simulink library "dsdc"  (Simulink 8.1)
settings: Solver=ode1  StartTime=0.0  StopTime=Inf  FixedStep=0.001  RelTol=1e-3
PostLoadFcn:
  | , if any(exist('dsrtsu_mdlpostloadfcn', 'file') == [2, 3, 6]), try dsrtsu_mdlpostloadfcn('Execute', bdroot); catch fprintf('Error in PostLoadFcn (dsrtsu_mdlpostloadfcn) for model "%s":\n %s\n', bdroot, lasterr); end, end,
undefined symbols (not defined in the file or in its folder): KJUD_EarlyTtcDelay_ms, KJUD_LateTtcDelay_ms, KJUD_NormalTtcDelay_ms
settings Model: DSRTSU_INTERNAL_RTI_VER=450  DSRTSU_INTERNAL_RTI_TYPE=rti1401  RTICANMMDATA=struct('GeneralSetupData',struct('modelroot','C:\Users\idiada\Desktop\HAITEC_Taiwan\trunk\AdasDragon\software\sw_development\arch\app\jud','generalsettings',struct('filesettings',struct('destfolder',struct('Name','RTICANMM_FILES','Check',1),'buildfolder',struct('Name','.','Check',1),'AbsDestfolder',struct('Name','C:\Users\idiada\Desktop\HAITEC_Taiwan\trunk\AdasDragon\software\sw_development\arch\app\jud\RTICANMM_FILES'),'AbsBuildfolder',struct('Name','C:\Users\idiada\Desktop\HAITEC_Taiwan\trunk\AdasDragon\software\sw_development\arch\app\jud'))),'options',struct('addpaths',1,'rmpaths',1,'addtrcexclusion',logical(1),'cannavigator',struct('checkmonitoring',0),'show_usrtrc',0,'use_usrtrc',0),'advanced',struct('options',[1 1 1 1 1 1 1 1 1 1 1 1 1 1 1 1 1 1 1 1 1 1 1 1 1 1 1 1 1 1 1 1 1 1 1 1 1 1 1 1 1 1 1 1 1 1 1 1 1 1 1 1 1 1 1 1 1 1 1 1 1 1 1 1 1 1 1 1 1 1 1 1 1 1 1 1 1 1 1 1 1 1 1 1 1 1 1 1 1 1 1 1 1 1 1 1 1 1 1 1]),'MPSetup',{{}},'modelname','dsdc','block','dsdc'))  DSRTSU_INTERNAL_RTIFPGA=40  Creator=idiada  LastModifiedBy=idiada

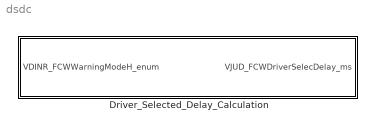
== system dsdc ==
  Driver_Selected_Delay_Calculation : Subsystem

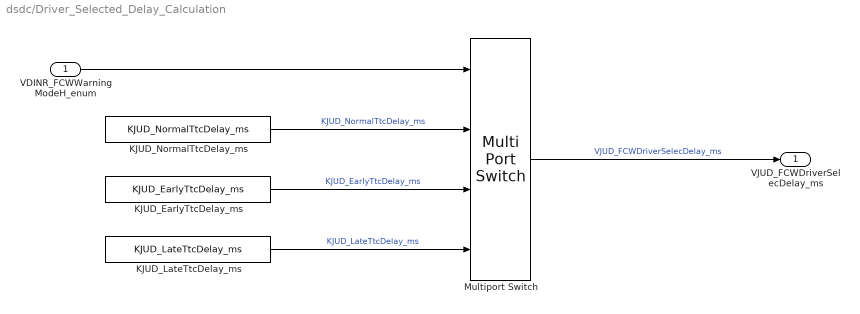
== system dsdc/Driver_Selected_Delay_Calculation ==
  VDINR_FCWWarningModeH_enum : Inport
  KJUD_EarlyTtcDelay_ms : Constant  Value=KJUD_EarlyTtcDelay_ms  OutDataTypeStr=single
  KJUD_LateTtcDelay_ms : Constant  Value=KJUD_LateTtcDelay_ms  OutDataTypeStr=single
  KJUD_NormalTtcDelay_ms : Constant  Value=KJUD_NormalTtcDelay_ms  OutDataTypeStr=single
  Multiport Switch : MultiPortSwitch  DataPortOrder=Zero-based contiguous
  VJUD_FCWDriverSelecDelay_ms : Outport
  wires:
  VDINR_FCWWarningModeH_enum/1 -> Multiport Switch/1
  Multiport Switch/1 -> VJUD_FCWDriverSelecDelay_ms/1  "VJUD_FCWDriverSelecDelay_ms"
  KJUD_NormalTtcDelay_ms/1 -> Multiport Switch/2  "KJUD_NormalTtcDelay_ms"
  KJUD_EarlyTtcDelay_ms/1 -> Multiport Switch/3  "KJUD_EarlyTtcDelay_ms"
  KJUD_LateTtcDelay_ms/1 -> Multiport Switch/4  "KJUD_LateTtcDelay_ms"
